simulink model "ctrl_studentmclab"  (R2015a)
settings: Solver=ode4  StartTime=0.0  StopTime=inf  FixedStep=0.01  RelTol=1e-3
(part 3 of 3)

== system ctrl_studentmclab/Observer/eta_hat_ut ==
  In1 : Inport
  Demux1 : Demux  Outputs=3
  psi_hat : S-Function  Priority=1  FunctionName=NIVeriStandIO  Parameters=width dtype portnum stime stype btype  mask(NI VeriStand Outport){portnum=1, width=-1, stime=-1, dtype=auto, stype=auto, btype=0}
      mask prompts: portnum "Port number:"; width "Port dimensions (-1 for dynamically sized):"; stime "Sample time (-1 for inherited):"; dtype "Data type:"; stype "Signal type:"; btype "Block type:"
      mask help: Use this outport on any level of nested subsystems to allow NI VeriStand software to map signals to it.
      mask init:
      | NIVeriStandIO_init;
      settings: CopyFcn=NIVeriStand_MDL_functions('', 'IO_copy');  DeleteFcn=NIVeriStand_MDL_functions('', 'IO_delete');  MoveFcn=set_param(gcb, 'Mask', 'on');
      mask Callback portnum: NIVeriStand_MDL_functions('', 'IO_setportnum');
      mask TypeOptions dtype: auto | double | single | int8 | uint8 | int16 | uint16 | int32 | uint32 | boolean
      mask Callback dtype: NIVeriStand_MDL_functions('', 'IO_booleansignal');
      mask TypeOptions stype: auto | real | complex
      mask Display:
      | patch([-x x], [-y y], [.90980 .81960 .32156]);
      | plot([xrad -x x xrad], [yrad -y y yrad]);
      | fprintf('NI Out%d', portnum);
  x_hat : S-Function  Priority=2  FunctionName=NIVeriStandIO  Parameters=width dtype portnum stime stype btype  mask(NI VeriStand Outport){portnum=2, width=-1, stime=-1, dtype=auto, stype=auto, btype=0}
      mask prompts: portnum "Port number:"; width "Port dimensions (-1 for dynamically sized):"; stime "Sample time (-1 for inherited):"; dtype "Data type:"; stype "Signal type:"; btype "Block type:"
      mask help: Use this outport on any level of nested subsystems to allow NI VeriStand software to map signals to it.
      mask init:
      | NIVeriStandIO_init;
      settings: CopyFcn=NIVeriStand_MDL_functions('', 'IO_copy');  DeleteFcn=NIVeriStand_MDL_functions('', 'IO_delete');  MoveFcn=set_param(gcb, 'Mask', 'on');
      mask Callback portnum: NIVeriStand_MDL_functions('', 'IO_setportnum');
      mask TypeOptions dtype: auto | double | single | int8 | uint8 | int16 | uint16 | int32 | uint32 | boolean
      mask Callback dtype: NIVeriStand_MDL_functions('', 'IO_booleansignal');
      mask TypeOptions stype: auto | real | complex
      mask Display:
      | patch([-x x], [-y y], [.90980 .81960 .32156]);
      | plot([xrad -x x xrad], [yrad -y y yrad]);
      | fprintf('NI Out%d', portnum);
  y_hat : S-Function  Priority=3  FunctionName=NIVeriStandIO  Parameters=width dtype portnum stime stype btype  mask(NI VeriStand Outport){portnum=3, width=-1, stime=-1, dtype=auto, stype=auto, btype=0}
      mask prompts: portnum "Port number:"; width "Port dimensions (-1 for dynamically sized):"; stime "Sample time (-1 for inherited):"; dtype "Data type:"; stype "Signal type:"; btype "Block type:"
      mask help: Use this outport on any level of nested subsystems to allow NI VeriStand software to map signals to it.
      mask init:
      | NIVeriStandIO_init;
      settings: CopyFcn=NIVeriStand_MDL_functions('', 'IO_copy');  DeleteFcn=NIVeriStand_MDL_functions('', 'IO_delete');  MoveFcn=set_param(gcb, 'Mask', 'on');
      mask Callback portnum: NIVeriStand_MDL_functions('', 'IO_setportnum');
      mask TypeOptions dtype: auto | double | single | int8 | uint8 | int16 | uint16 | int32 | uint32 | boolean
      mask Callback dtype: NIVeriStand_MDL_functions('', 'IO_booleansignal');
      mask TypeOptions stype: auto | real | complex
      mask Display:
      | patch([-x x], [-y y], [.90980 .81960 .32156]);
      | plot([xrad -x x xrad], [yrad -y y yrad]);
      | fprintf('NI Out%d', portnum);
  wires:
  Demux1/3 -> psi_hat/1
  Demux1/1 -> x_hat/1
  Demux1/2 -> y_hat/1
  In1/1 -> Demux1/1

== system ctrl_studentmclab/Observer/nu_hat_ut ==
  In1 : Inport
  Demux1 : Demux  Outputs=3
  r_hat : S-Function  Priority=1  FunctionName=NIVeriStandIO  Parameters=width dtype portnum stime stype btype  mask(NI VeriStand Outport){portnum=1, width=-1, stime=-1, dtype=auto, stype=auto, btype=0}
      mask prompts: portnum "Port number:"; width "Port dimensions (-1 for dynamically sized):"; stime "Sample time (-1 for inherited):"; dtype "Data type:"; stype "Signal type:"; btype "Block type:"
      mask help: Use this outport on any level of nested subsystems to allow NI VeriStand software to map signals to it.
      mask init:
      | NIVeriStandIO_init;
      settings: CopyFcn=NIVeriStand_MDL_functions('', 'IO_copy');  DeleteFcn=NIVeriStand_MDL_functions('', 'IO_delete');  MoveFcn=set_param(gcb, 'Mask', 'on');
      mask Callback portnum: NIVeriStand_MDL_functions('', 'IO_setportnum');
      mask TypeOptions dtype: auto | double | single | int8 | uint8 | int16 | uint16 | int32 | uint32 | boolean
      mask Callback dtype: NIVeriStand_MDL_functions('', 'IO_booleansignal');
      mask TypeOptions stype: auto | real | complex
      mask Display:
      | patch([-x x], [-y y], [.90980 .81960 .32156]);
      | plot([xrad -x x xrad], [yrad -y y yrad]);
      | fprintf('NI Out%d', portnum);
  u_hat : S-Function  Priority=2  FunctionName=NIVeriStandIO  Parameters=width dtype portnum stime stype btype  mask(NI VeriStand Outport){portnum=2, width=-1, stime=-1, dtype=auto, stype=auto, btype=0}
      mask prompts: portnum "Port number:"; width "Port dimensions (-1 for dynamically sized):"; stime "Sample time (-1 for inherited):"; dtype "Data type:"; stype "Signal type:"; btype "Block type:"
      mask help: Use this outport on any level of nested subsystems to allow NI VeriStand software to map signals to it.
      mask init:
      | NIVeriStandIO_init;
      settings: CopyFcn=NIVeriStand_MDL_functions('', 'IO_copy');  DeleteFcn=NIVeriStand_MDL_functions('', 'IO_delete');  MoveFcn=set_param(gcb, 'Mask', 'on');
      mask Callback portnum: NIVeriStand_MDL_functions('', 'IO_setportnum');
      mask TypeOptions dtype: auto | double | single | int8 | uint8 | int16 | uint16 | int32 | uint32 | boolean
      mask Callback dtype: NIVeriStand_MDL_functions('', 'IO_booleansignal');
      mask TypeOptions stype: auto | real | complex
      mask Display:
      | patch([-x x], [-y y], [.90980 .81960 .32156]);
      | plot([xrad -x x xrad], [yrad -y y yrad]);
      | fprintf('NI Out%d', portnum);
  v_hat : S-Function  Priority=3  FunctionName=NIVeriStandIO  Parameters=width dtype portnum stime stype btype  mask(NI VeriStand Outport){portnum=3, width=-1, stime=-1, dtype=auto, stype=auto, btype=0}
      mask prompts: portnum "Port number:"; width "Port dimensions (-1 for dynamically sized):"; stime "Sample time (-1 for inherited):"; dtype "Data type:"; stype "Signal type:"; btype "Block type:"
      mask help: Use this outport on any level of nested subsystems to allow NI VeriStand software to map signals to it.
      mask init:
      | NIVeriStandIO_init;
      settings: CopyFcn=NIVeriStand_MDL_functions('', 'IO_copy');  DeleteFcn=NIVeriStand_MDL_functions('', 'IO_delete');  MoveFcn=set_param(gcb, 'Mask', 'on');
      mask Callback portnum: NIVeriStand_MDL_functions('', 'IO_setportnum');
      mask TypeOptions dtype: auto | double | single | int8 | uint8 | int16 | uint16 | int32 | uint32 | boolean
      mask Callback dtype: NIVeriStand_MDL_functions('', 'IO_booleansignal');
      mask TypeOptions stype: auto | real | complex
      mask Display:
      | patch([-x x], [-y y], [.90980 .81960 .32156]);
      | plot([xrad -x x xrad], [yrad -y y yrad]);
      | fprintf('NI Out%d', portnum);
  wires:
  Demux1/3 -> r_hat/1
  Demux1/1 -> u_hat/1
  Demux1/2 -> v_hat/1
  In1/1 -> Demux1/1

== system ctrl_studentmclab/tau to real ship (only use in MCLab)/To thruster of real ship ==
  u to thrusters : Inport
  control input u exceeds bounds : S-Function  Priority=8  FunctionName=NIVeriStandIO  Parameters=width dtype portnum stime stype btype  mask(NI VeriStand Outport){portnum=8, width=-1, stime=-1, dtype=auto, stype=auto, btype=0}
      mask prompts: portnum "Port number:"; width "Port dimensions (-1 for dynamically sized):"; stime "Sample time (-1 for inherited):"; dtype "Data type:"; stype "Signal type:"; btype "Block type:"
      mask help: Use this outport on any level of nested subsystems to allow NI VeriStand software to map signals to it.
      mask init:
      | NIVeriStandIO_init;
      settings: CopyFcn=NIVeriStand_MDL_functions('', 'IO_copy');  DeleteFcn=NIVeriStand_MDL_functions('', 'IO_delete');  MoveFcn=set_param(gcb, 'Mask', 'on');
      mask Callback portnum: NIVeriStand_MDL_functions('', 'IO_setportnum');
      mask TypeOptions dtype: auto | double | single | int8 | uint8 | int16 | uint16 | int32 | uint32 | boolean
      mask Callback dtype: NIVeriStand_MDL_functions('', 'IO_booleansignal');
      mask TypeOptions stype: auto | real | complex
      mask Display:
      | patch([-x x], [-y y], [.90980 .81960 .32156]);
      | plot([xrad -x x xrad], [yrad -y y yrad]);
      | fprintf('NI Out%d', portnum);
  control limit checking : MATLAB Function  TreatAsAtomicUnit=on
  u : Subsystem
  wires:
  control limit checking/1(fault) -> control input u exceeds bounds/1
  u to thrusters/1 -> control limit checking/1(u), u/1(u)

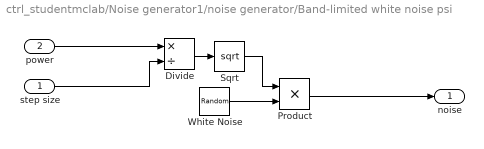
== system ctrl_studentmclab/Noise generator1/noise generator/Band-limited white noise psi ==
  step size : Inport
  power : Inport  Port=2
  Divide : Product  Inputs=*/
  Product : Product
  Sqrt : Sqrt  SaturateOnIntegerOverflow=on
  White Noise : RandomNumber  DisableCoverage=on  Seed=9025
  noise : Outport
  wires:
  White Noise/1 -> Product/2
  Product/1 -> noise/1
  step size/1 -> Divide/2
  Divide/1 -> Sqrt/1
  Sqrt/1 -> Product/1
  power/1 -> Divide/1

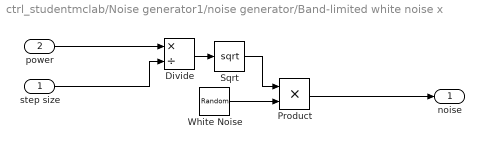
== system ctrl_studentmclab/Noise generator1/noise generator/Band-limited white noise x ==
  step size : Inport
  power : Inport  Port=2
  Divide : Product  Inputs=*/
  Product : Product
  Sqrt : Sqrt  SaturateOnIntegerOverflow=on
  White Noise : RandomNumber  DisableCoverage=on  Seed=9024
  noise : Outport
  wires:
  White Noise/1 -> Product/2
  Product/1 -> noise/1
  step size/1 -> Divide/2
  Divide/1 -> Sqrt/1
  Sqrt/1 -> Product/1
  power/1 -> Divide/1

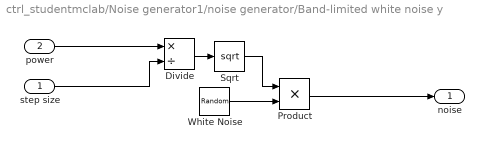
== system ctrl_studentmclab/Noise generator1/noise generator/Band-limited white noise y ==
  step size : Inport
  power : Inport  Port=2
  Divide : Product  Inputs=*/
  Product : Product
  Sqrt : Sqrt  SaturateOnIntegerOverflow=on
  White Noise : RandomNumber  DisableCoverage=on  Seed=123
  noise : Outport
  wires:
  White Noise/1 -> Product/2
  Product/1 -> noise/1
  step size/1 -> Divide/2
  Divide/1 -> Sqrt/1
  Sqrt/1 -> Product/1
  power/1 -> Divide/1

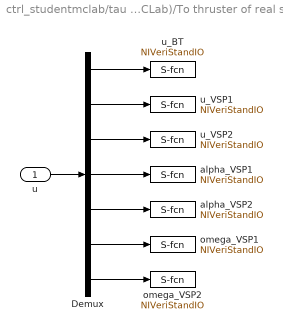
== system ctrl_studentmclab/tau to real ship (only use in MCLab)/To thruster of real ship/u ==
  u : Inport
  Demux : Demux  Outputs=7
  alpha_VSP1 : S-Function  Priority=4  FunctionName=NIVeriStandIO  Parameters=width dtype portnum stime stype btype  mask(NI VeriStand Outport){portnum=4, width=-1, stime=-1, dtype=auto, stype=auto, btype=0}
      mask prompts: portnum "Port number:"; width "Port dimensions (-1 for dynamically sized):"; stime "Sample time (-1 for inherited):"; dtype "Data type:"; stype "Signal type:"; btype "Block type:"
      mask help: Use this outport on any level of nested subsystems to allow NI VeriStand software to map signals to it.
      mask init:
      | NIVeriStandIO_init;
      settings: CopyFcn=NIVeriStand_MDL_functions('', 'IO_copy');  DeleteFcn=NIVeriStand_MDL_functions('', 'IO_delete');  MoveFcn=set_param(gcb, 'Mask', 'on');
      mask Callback portnum: NIVeriStand_MDL_functions('', 'IO_setportnum');
      mask TypeOptions dtype: auto | double | single | int8 | uint8 | int16 | uint16 | int32 | uint32 | boolean
      mask Callback dtype: NIVeriStand_MDL_functions('', 'IO_booleansignal');
      mask TypeOptions stype: auto | real | complex
      mask Display:
      | patch([-x x], [-y y], [.90980 .81960 .32156]);
      | plot([xrad -x x xrad], [yrad -y y yrad]);
      | fprintf('NI Out%d', portnum);
  alpha_VSP2 : S-Function  Priority=1  FunctionName=NIVeriStandIO  Parameters=width dtype portnum stime stype btype  mask(NI VeriStand Outport){portnum=1, width=-1, stime=-1, dtype=auto, stype=auto, btype=0}
      mask prompts: portnum "Port number:"; width "Port dimensions (-1 for dynamically sized):"; stime "Sample time (-1 for inherited):"; dtype "Data type:"; stype "Signal type:"; btype "Block type:"
      mask help: Use this outport on any level of nested subsystems to allow NI VeriStand software to map signals to it.
      mask init:
      | NIVeriStandIO_init;
      settings: CopyFcn=NIVeriStand_MDL_functions('', 'IO_copy');  DeleteFcn=NIVeriStand_MDL_functions('', 'IO_delete');  MoveFcn=set_param(gcb, 'Mask', 'on');
      mask Callback portnum: NIVeriStand_MDL_functions('', 'IO_setportnum');
      mask TypeOptions dtype: auto | double | single | int8 | uint8 | int16 | uint16 | int32 | uint32 | boolean
      mask Callback dtype: NIVeriStand_MDL_functions('', 'IO_booleansignal');
      mask TypeOptions stype: auto | real | complex
      mask Display:
      | patch([-x x], [-y y], [.90980 .81960 .32156]);
      | plot([xrad -x x xrad], [yrad -y y yrad]);
      | fprintf('NI Out%d', portnum);
  omega_VSP1 : S-Function  Priority=2  FunctionName=NIVeriStandIO  Parameters=width dtype portnum stime stype btype  mask(NI VeriStand Outport){portnum=2, width=-1, stime=-1, dtype=auto, stype=auto, btype=0}
      mask prompts: portnum "Port number:"; width "Port dimensions (-1 for dynamically sized):"; stime "Sample time (-1 for inherited):"; dtype "Data type:"; stype "Signal type:"; btype "Block type:"
      mask help: Use this outport on any level of nested subsystems to allow NI VeriStand software to map signals to it.
      mask init:
      | NIVeriStandIO_init;
      settings: CopyFcn=NIVeriStand_MDL_functions('', 'IO_copy');  DeleteFcn=NIVeriStand_MDL_functions('', 'IO_delete');  MoveFcn=set_param(gcb, 'Mask', 'on');
      mask Callback portnum: NIVeriStand_MDL_functions('', 'IO_setportnum');
      mask TypeOptions dtype: auto | double | single | int8 | uint8 | int16 | uint16 | int32 | uint32 | boolean
      mask Callback dtype: NIVeriStand_MDL_functions('', 'IO_booleansignal');
      mask TypeOptions stype: auto | real | complex
      mask Display:
      | patch([-x x], [-y y], [.90980 .81960 .32156]);
      | plot([xrad -x x xrad], [yrad -y y yrad]);
      | fprintf('NI Out%d', portnum);
  omega_VSP2 : S-Function  Priority=3  FunctionName=NIVeriStandIO  Parameters=width dtype portnum stime stype btype  mask(NI VeriStand Outport){portnum=3, width=-1, stime=-1, dtype=auto, stype=auto, btype=0}
      mask prompts: portnum "Port number:"; width "Port dimensions (-1 for dynamically sized):"; stime "Sample time (-1 for inherited):"; dtype "Data type:"; stype "Signal type:"; btype "Block type:"
      mask help: Use this outport on any level of nested subsystems to allow NI VeriStand software to map signals to it.
      mask init:
      | NIVeriStandIO_init;
      settings: CopyFcn=NIVeriStand_MDL_functions('', 'IO_copy');  DeleteFcn=NIVeriStand_MDL_functions('', 'IO_delete');  MoveFcn=set_param(gcb, 'Mask', 'on');
      mask Callback portnum: NIVeriStand_MDL_functions('', 'IO_setportnum');
      mask TypeOptions dtype: auto | double | single | int8 | uint8 | int16 | uint16 | int32 | uint32 | boolean
      mask Callback dtype: NIVeriStand_MDL_functions('', 'IO_booleansignal');
      mask TypeOptions stype: auto | real | complex
      mask Display:
      | patch([-x x], [-y y], [.90980 .81960 .32156]);
      | plot([xrad -x x xrad], [yrad -y y yrad]);
      | fprintf('NI Out%d', portnum);
  u_BT : S-Function  Priority=5  FunctionName=NIVeriStandIO  Parameters=width dtype portnum stime stype btype  mask(NI VeriStand Outport){portnum=5, width=-1, stime=-1, dtype=auto, stype=auto, btype=0}
      mask prompts: portnum "Port number:"; width "Port dimensions (-1 for dynamically sized):"; stime "Sample time (-1 for inherited):"; dtype "Data type:"; stype "Signal type:"; btype "Block type:"
      mask help: Use this outport on any level of nested subsystems to allow NI VeriStand software to map signals to it.
      mask init:
      | NIVeriStandIO_init;
      settings: CopyFcn=NIVeriStand_MDL_functions('', 'IO_copy');  DeleteFcn=NIVeriStand_MDL_functions('', 'IO_delete');  MoveFcn=set_param(gcb, 'Mask', 'on');
      mask Callback portnum: NIVeriStand_MDL_functions('', 'IO_setportnum');
      mask TypeOptions dtype: auto | double | single | int8 | uint8 | int16 | uint16 | int32 | uint32 | boolean
      mask Callback dtype: NIVeriStand_MDL_functions('', 'IO_booleansignal');
      mask TypeOptions stype: auto | real | complex
      mask Display:
      | patch([-x x], [-y y], [.90980 .81960 .32156]);
      | plot([xrad -x x xrad], [yrad -y y yrad]);
      | fprintf('NI Out%d', portnum);
  u_VSP1 : S-Function  Priority=6  FunctionName=NIVeriStandIO  Parameters=width dtype portnum stime stype btype  mask(NI VeriStand Outport){portnum=6, width=-1, stime=-1, dtype=auto, stype=auto, btype=0}
      mask prompts: portnum "Port number:"; width "Port dimensions (-1 for dynamically sized):"; stime "Sample time (-1 for inherited):"; dtype "Data type:"; stype "Signal type:"; btype "Block type:"
      mask help: Use this outport on any level of nested subsystems to allow NI VeriStand software to map signals to it.
      mask init:
      | NIVeriStandIO_init;
      settings: CopyFcn=NIVeriStand_MDL_functions('', 'IO_copy');  DeleteFcn=NIVeriStand_MDL_functions('', 'IO_delete');  MoveFcn=set_param(gcb, 'Mask', 'on');
      mask Callback portnum: NIVeriStand_MDL_functions('', 'IO_setportnum');
      mask TypeOptions dtype: auto | double | single | int8 | uint8 | int16 | uint16 | int32 | uint32 | boolean
      mask Callback dtype: NIVeriStand_MDL_functions('', 'IO_booleansignal');
      mask TypeOptions stype: auto | real | complex
      mask Display:
      | patch([-x x], [-y y], [.90980 .81960 .32156]);
      | plot([xrad -x x xrad], [yrad -y y yrad]);
      | fprintf('NI Out%d', portnum);
  u_VSP2 : S-Function  Priority=7  FunctionName=NIVeriStandIO  Parameters=width dtype portnum stime stype btype  mask(NI VeriStand Outport){portnum=7, width=-1, stime=-1, dtype=auto, stype=auto, btype=0}
      mask prompts: portnum "Port number:"; width "Port dimensions (-1 for dynamically sized):"; stime "Sample time (-1 for inherited):"; dtype "Data type:"; stype "Signal type:"; btype "Block type:"
      mask help: Use this outport on any level of nested subsystems to allow NI VeriStand software to map signals to it.
      mask init:
      | NIVeriStandIO_init;
      settings: CopyFcn=NIVeriStand_MDL_functions('', 'IO_copy');  DeleteFcn=NIVeriStand_MDL_functions('', 'IO_delete');  MoveFcn=set_param(gcb, 'Mask', 'on');
      mask Callback portnum: NIVeriStand_MDL_functions('', 'IO_setportnum');
      mask TypeOptions dtype: auto | double | single | int8 | uint8 | int16 | uint16 | int32 | uint32 | boolean
      mask Callback dtype: NIVeriStand_MDL_functions('', 'IO_booleansignal');
      mask TypeOptions stype: auto | real | complex
      mask Display:
      | patch([-x x], [-y y], [.90980 .81960 .32156]);
      | plot([xrad -x x xrad], [yrad -y y yrad]);
      | fprintf('NI Out%d', portnum);
  wires:
  u/1 -> Demux/1
  Demux/1 -> u_BT/1
  Demux/2 -> u_VSP1/1
  Demux/3 -> u_VSP2/1
  Demux/4 -> alpha_VSP1/1
  Demux/5 -> alpha_VSP2/1
  Demux/6 -> omega_VSP1/1
  Demux/7 -> omega_VSP2/1

== matlab function ctrl_studentmclab/tau to real ship (only use in MCLab)/Full thrust allocation ==
  data: X_d input; Y_d input; u_BT output; N_d input; u_VSP output; alpha_VSP output; VSP_on input; omega_VSP output
function [u_BT,u_VSP,alpha_VSP,omega_VSP]= fcn(X_d,Y_d,N_d, VSP_on)

% Forces and moments vector
tau = [X_d
       Y_d
       N_d];

% Extended thrust configuration matrix
l_VSP = -0.4575;
l_BT  = 0.3875;
T = [1 0     0
     0 1     1
     0 l_VSP l_BT];

% Extended thrust coefficient matrix
F_max_VSP = 1.165;
F_max_BT  = 2.629;
K = [F_max_VSP 0         0
     0         F_max_VSP 0
     0         0         F_max_BT];

% tau = T*K*u inverse
u = K\(T\tau);

u_BT      = u(3);

u_VSP_x   = u(1);
u_VSP_y   = u(2);
u_VSP     = sqrt(u_VSP_x^2 + u_VSP_y^2);
alpha_VSP = atan2(u_VSP_y,u_VSP_x);

if VSP_on
    omega_VSP = 0.3;
else
    omega_VSP = 0;
end

== matlab function ctrl_studentmclab/tau to real ship (only use in MCLab)/To thruster of real ship/control limit checking ==
  data: u input; fault output
function fault= fcn(u)
u_BT       = u(1);
u_VSP1     = u(2);
u_VSP2     = u(3);
alpha_VSP1 = u(4);
alpha_VSP2 = u(5);
omega_VSP1 = u(6);
omega_VSP2 = u(7);

OK = -1  <= u_BT       & u_BT       <= 1  & ...
     0   <= u_VSP1     & u_VSP1     <= 1  & ...
     0   <= u_VSP2     & u_VSP2     <= 1  & ...
     -pi <= alpha_VSP1 & alpha_VSP1 <= pi & ...
     -pi <= alpha_VSP2 & alpha_VSP2 <= pi & ...
     -1  <= omega_VSP1 & omega_VSP1 <= 1  & ...
     -1  <= omega_VSP2 & omega_VSP2 <= 1  ;
 
fault = ~OK;

== matlab function ctrl_studentmclab/tau to real ship (only use in MCLab)/Limited allocation: VSP only  in surge and BT only in yaw ==
  data: X_VSP input; u_BT output; N_BT input; u_VSP output; alpha_VSP output; omega_VSP output
function [u_BT,u_VSP,alpha_VSP,omega_VSP]= fcn(X_VSP,N_BT)

l_BT     = 0.3875;
F_max_BT = 2.629;
u_BT     = N_BT/(l_BT*F_max_BT);

omega_VSP = 0.3;
F_max_VSP = 1.165;
u_VSP     = abs(X_VSP)/(2*F_max_VSP);
alpha_VSP = pi*(X_VSP<=0); % 0 if positive X_VSP, pi if negative

== matlab function ctrl_studentmclab/Noise generator1/Downsample	signal/MATLAB Function ==
  data: f input; h input; i input; count output
function count = fcn(f,h,i)
%#codegen
sampling_time = 1/f;
if (i+1)*h >= sampling_time
    count = 0;
else
    count = i+1;
end

== matlab function ctrl_studentmclab/Noise generator1/Sample & hold/MATLAB Function1 ==
  data: counter input; input input; hold input; output output
function output = fcn(counter,input,hold)
%#codegen

if counter == 0
    output = input;
else
    output = hold;
end

== matlab function ctrl_studentmclab/Observer/D ==
  data: nu input; D output
function D = fcn(nu)

d11 = 0.6555-0.354*abs(nu(1))+3.787*(nu(1))^2; 
d22 = 1.33+2.776*abs(nu(2))+64.91*(nu(2))^2+0.805*abs(nu(3)) ; 
d23 = 7.25+0.845*abs(nu(2))+3.45*abs(nu(3));
d32 = 0.2088*abs(nu(2))-0.130*abs(nu(3));
d33 = 1.9-0.08*abs(nu(2))+0.75*abs(nu(3));

D=[d11 0    0
   0   d22  d23
   0   d32  d33];

== matlab function ctrl_studentmclab/Observer/L1/MATLAB Function ==
  data: u input; y output
function y = fcn(u)
y = diag([u(1),u(2),u(3)]);

== matlab function ctrl_studentmclab/DP-system/Ellipsoidal path ==
  data: s input; c input; eta_v output size=11; r input; U_ref input; psi input
function eta_v = fcn(s,c,r,U_ref,psi)

eta_d = [c(1) + r(1)*cos(2*pi*s)
         c(2) + r(2)*sin(2*pi*s)
         atan2(-r(2)*cos(2*pi*s),r(1)*sin(2*pi*s))];

%wrapping psi_d     
persistent k;
k=0;				

if abs((eta_d(3)+(2*pi*k))-(psi)) > pi
   if (psi) < eta_d(3)+(2*pi*k)
       k = k-1;
   elseif (psi) > eta_d(3)+(2*pi*k)
       k = k+1;
   end
end 
eta_d(3)=eta_d(3)+(2*pi*k);
     
     
eta_ds = 2*pi*[-r(1)*sin(2*pi*s)
                r(2)*cos(2*pi*s)
               (-r(1)*r(2))/(r(2)^2*cos(2*pi*s)^2 + r(1)^2*sin(2*pi*s)^2)];

eta_dss = (2*pi)^2*[-r(1)*cos(2*pi*s)
                     -r(2)*sin(2*pi*s)
                     (4*r(2)*r(1)*(r(2)^2 - r(1)^2)*sin(2*2*pi*s))/(r(2)^2 + r(1)^2 + r(2)^2*cos(2*2*pi*s) - r(1)^2*cos(2*2*pi*s))^2];
     
     
U_s = U_ref/(sqrt(r(1)^2 * sin(2*pi*s)^2 + r(2)^2 * cos(2*pi*s)^2));

U_ss = -U_ref*(r(1)^2*sin(2*pi*s)*(2*pi)^3*cos(2*pi*s)-r(2)^2*cos(2*pi*s)*(2*pi)^3*sin(2*pi*s))/...
    ((2*pi*-r(1)*sin(2*pi*s))^2 + (r(2)*cos(2*pi*s)*2*pi)^2)^1.5;

eta_v = [eta_d; eta_ds; eta_dss ; U_s; U_ss];

== matlab function ctrl_studentmclab/Observer/L2/MATLAB Function ==
  data: u input; y output
function y = fcn(u)
y = diag([u(1),u(2),u(3)]);

== matlab function ctrl_studentmclab/DP-system/controller ==
  data: z1 input; z2 input; s_dot input; a_1 output; eta_v input; nu input; tau output; Kd input; D1 output; z11 output; ma output; Kdz output
function [a_1, tau,D1,z11,ma,Kdz] = fcn(z1,z2,s_dot,eta_v,nu,Kd)
%Kinetics
u   = nu(1);
v   = nu(2);
r   = nu(3);
% MATRICES
m    = 14.79;   
I_z  =  1.76;  
x_g = 0.0375;       
% Added mass
X_ud  =     -2.0;						% Table B.1
Y_vd =     -1.0;	N_vd =    -0.0;		% Table B.1 guestimate
Y_rd =      -0.0;	N_rd =    -1.0;		% Table B.1

% Total mass matrix
m_11 = m-X_ud;
m_22 = m-Y_vd;
m_23 = m*x_g-Y_rd;
m_32 = m*x_g-N_vd;
m_33 = I_z-N_rd;

M    = [m_11 0    0
        0    m_22 m_23
        0    m_32 m_33];
	
% Damping coefficients
% Comments at the end of the lines indicate the old values used.
X_u		= -0.6555;		X_v		= 0;
X_uu 	= 0.3545;		X_vv	= -2.443;
X_uuu 	= -3.787;		X_vvv	= 0;
Y_v		= -1.33;    	Y_r		= -7.250; % Y_r
Y_vv	= -2.776;		Y_rr	= -3.450; % Y_rr
Y_vvv	= -64.91;		Y_rrr	= 0;
Y_rv	= -0.805;		Y_vr	= -0.845; % Y_rv, Y_vr
N_v		= 0;			N_r		= -1.900; % N_r
N_vv	= -0.2088;		N_rr	= -0.750; % N_rr
N_vvv	= 0;			N_rrr	= 0;
N_rv	= 0.130;		N_vr	= 0.080; % N_rv, N_vr

% Correolis matrix
c_13 = -(m-Y_vd)*v-(m*x_g-Y_rd)*r;
c_23 = (m-X_ud)*u;
C    = [0     0     c_13
        0     0     c_23
        -c_13 -c_23 0   ];

% Assembly of the damping matrix
d_11 = -X_u - X_uu*u - X_uuu*u^2;
d_22 = -Y_v - Y_vv*v - Y_vvv*v^2 - Y_rv*abs(r);
d_33 = -N_r - N_rr*abs(r) - N_rrr*r^2 - N_vr*abs(v); % using abs(r)

d_12 = -X_v - X_vv*v - X_vvv*v^2;
d_23 = -Y_r - Y_rr*abs(r) - Y_rrr*r^2 - Y_vr*abs(v);
d_32 = -N_v - N_vv*v - N_vvv*v^2 - N_rv*abs(r);

D    = [d_11 d_12 0
        0    d_22 d_23
        0    d_32 d_33];

    

%Eta_d derivatives and U_s
eta     = eta_v(1:3);
eta_ds  = eta_v(4:6);
eta_dss = eta_v(7:9);
U_s     = eta_v(10);
U_ss    = eta_v(11);
%Rotation matrix and derivative
R = [cos(eta(3)) -sin(eta(3)) 0
     sin(eta(3))  cos(eta(3)) 0
     0            0           1];
 
S = [0     -eta(3) 0
     eta(3)   0    0
     0        0    0]; 
 
%Gain matrices 
Kp = diag([0.2,0.2,0.1]);
%Kd = diag([25 15 30]);

%Controller alpha 1
a_1 = -Kp*z1 +R'*eta_ds*U_s;


%Alpha derivative
a_t = -Kp*(-S*z1+nu)-S*R'*eta_ds*U_s;
a_s = -Kp*R'*eta_ds+R'*eta_dss*U_s+R'*eta_ds*U_ss;
a_dot = a_t + a_s.*s_dot;

%Controller tau - C removed
tau = D*nu- z1 + M*a_dot - Kd*z2;
D1 = D*nu;
z11 = z1;
ma = M*a_dot;
Kdz = Kd*z2;
%tau = a_1;
%tau = [tau(1);tau(2);tau(3)];

== matlab function ctrl_studentmclab/DP-system/Straight -line  ==
  data: eta_0 input; eta_1 input; U_ref input; eta_v output size=11; s input
function eta_v = fcn(eta_0,eta_1,U_ref,s)

eta_d = [(eta_1(1)-eta_0(1))*s + eta_0(1)
         (eta_1(2)-eta_0(2))*s + eta_0(2) 
         atan((eta_1(2)-eta_0(2))/(eta_1(1)-eta_0(1)))];
     
eta_ds = [(eta_1(1)-eta_0(1))
          (eta_1(2)-eta_0(2))
          0];
eta_dss = [0; 0; 0];



     
U_s = U_ref / sqrt((eta_1(1)-eta_0(1))^2 + (eta_1(2)-eta_0(2))^2);

U_ss = 0;

 
eta_v = [eta_d; eta_ds; eta_dss ; U_s; U_ss];

== matlab function ctrl_studentmclab/DP-system/update law ==
  data: eta input; eta_v input; z1 input; my input; s_dot1 output size=1; temp input; i output
function [s_dot1,i] = fcn(eta,eta_v,z1,my,temp)

i = temp(1); 
s = temp(3); 
s_dot1 = temp(2);
%Getting vectors
eta_d   = eta_v(1:3);
eta_ds  = eta_v(4:6);
eta_dss = eta_v(7:9);
U_s     = eta_v(10);


R = [cos(eta(3)) -sin(eta(3)) 0
     sin(eta(3))  cos(eta(3)) 0
     0            0           1];

V1_s = -z1'*R'*eta_ds;



    s_dot1 = U_s - (my/norm(eta_ds))*V1_s;

if i == 0 
    
    if s > 1;
        i = 1; 
    end 
end 

if i == 1
    s_dot1 = -(U_s - (my/norm(eta_ds))*V1_s); 
    if s < 0;
        i = 0; 
    end 
end

== matlab function ctrl_studentmclab/DP-system/z1//z2 ==
  data: eta_v input; z1 output; eta input; nu input; alpha input; z2 output
function [z1,z2]  = fcn(eta_v,eta,nu,alpha)


eta_d1 = [eta_v(1);eta_v(2);eta_v(3)];
eta1 = [eta(1);eta(2);eta(3)];

R = [cos(eta(3)) -sin(eta(3)) 0
     sin(eta(3))  cos(eta(3)) 0
     0            0           1];
 
 z1 = R'*(eta1-eta_d1);
 
 z2 = nu - alpha;

== matlab function ctrl_studentmclab/Observer/L3/MATLAB Function ==
  data: u input; y output
function y = fcn(u)
y = diag([u(1),u(2),u(3)]);

== matlab function ctrl_studentmclab/Observer/Rotation matrix ==
  data: psi input; R output; RT output
function [R,RT] = fcn(psi)
R=[ cos(psi) -sin(psi) 0
    sin(psi) cos(psi)  0
    0        0         1];

RT=R';

== matlab function ctrl_studentmclab/DP-system/signal switch  ==
  data: straight input; signal output; swich input; ellipse input
function signal = fcn(straight,swich,ellipse)

signal = straight; 
if swich == 1
    signal = straight;
end

if swich == 2
    signal = ellipse;
end

== matlab function ctrl_studentmclab/DP-system/Kd/MATLAB Function ==
  data: u input; y output
function y = fcn(u)
y = diag([u(1),u(2),u(3)]);

== matlab function ctrl_studentmclab/DP-system/inputs ==
  data: eta input; eta_0 output; eta_d output; U_ref_l output; r output; c output; U_ref_e output; my output; s input
function [eta_0,eta_d,U_ref_l,r,c,U_ref_e,my]  = fcn(eta,s)
% i = temp1(1);  
% U_ref_l = temp1(2); 
eta_0 = [2 0];
eta_d = [4 2]; 
r = [7 7]; 
c = [0 0];  
U_max = 0.5; 
my = 0; 
dp = 0; % my må være null hvis dp = 1
U_ref_l = U_max/5;
U_ref_e = 0.05;


% % ikke dp i starten
% 
%     if i == 0
%         U_ref_l = U_max/5; 
%         if s > 1;
%             i = 1; 
%         end 
%     end 
% 
%     if i == 1
%         U_ref_l = -U_max/5;
%         if s < 0
%             i = 0; 
%         end
%     end 
% U_ref = U_ref_l;
% 
% % error = [0 0];
% % error(1) = eta(1) - eta_0(1);
% % error(2) = eta(2) - eta_0(2); 
% % DP i starten
% % if dp == 1 
% % if i == 0 
% %     if (abs(error(1)) < 0.01 && abs(error(2)) < 0.01)
% %     U_ref_l = U_max/5;
% %     i = 1; 
% %     end
% % end 
% % 
% % if i == 1
% %     if s >= 1
% %         U_ref_l = -U_max/5;
% %         i = 2; 
% %     end     
% % end
% % 
% % if i == 2
% %     if s <= 0 
% %         U_ref_l = U_max/5; 
% %         i = 1; 
% %     end 
% % end 
% % end
% 
% temp = [0 0];
% temp(1) = i; 
% temp(2) = U_ref_l;

== matlab function ctrl_studentmclab/Switch joystick and DP-system ==
  data: guidance input; signal output; swich input; joystick input
%% Function that takes in impulse button sigals [0,1] and sends out a 
% different signal depentent pn which button has been pressed

function signal = fcn(guidance,swich,joystick)

signal = [0;0;0]; 
if swich == 1
    signal = guidance;
end

if swich == 2
    signal = guidance;
end

if swich == 3
    signal = joystick;
end

== matlab function ctrl_studentmclab/joystick1/MATLAB Function ==
  data: x input; u output; y input
function u = fcn(x,y)

if abs(x) > 5 || abs(y) > 5
    u = 1; %wtf fiks 
else 
    u = 1;
end

== matlab function ctrl_studentmclab/joystick1/Thrust allocation ==
  data: X input; Y input; u_BT output; N input; u_VSP output; alpha_VSP output; VSP_on input; omega_VSP output
function [u_BT,u_VSP,alpha_VSP,omega_VSP]= fcn(X,Y,N, VSP_on)

% Forces and moments vector
tau = [X
       Y
       N];

% Extended thrust configuration matrix
l_VSP = -0.4575;
l_BT  = 0.3875;
T = [1 0     0
     0 1     1
     0 l_VSP l_BT];

% Extended thrust coefficient matrix
F_max_VSP = 1.165;
F_max_BT  = 2.629;
K = [F_max_VSP 0         0
     0         F_max_VSP 0
     0         0         F_max_BT];

% tau = T*K*u inverse
u = (T*K)\tau;

u_BT      = u(3);

u_VSP_x   = u(1);
u_VSP_y   = u(2);
u_VSP     = sqrt(u_VSP_x^2 + u_VSP_y^2);
alpha_VSP = atan2(u_VSP_y,u_VSP_x);

if VSP_on
    omega_VSP = 0.3;
else
    omega_VSP = 0;
end

== matlab function ctrl_studentmclab/signal dropout check /MATLAB Function ==
  data: u input; y output; v input; vecx1 input; vecx output; vecy1 input; vecy output; d output
function [y,vecx,vecy,d] = fcn(u,v,vecx1,vecy1) 
vecx = vecx1;
vecy = vecy1;
for i = 2:10
vecx(i) = vecx(i-1);
vecy(i) = vecy(i-1);
end
vecx(1) = u(1);
vecy(1) = u(2); 

d = 1; 
if (numel(unique(vecx)) == 1 || numel(unique(vecy)) == 1)
    y = v; 
    d = 0;
else
    y = u;
end

== matlab function ctrl_studentmclab/switch/Switch_function ==
  data: arrows input; switch_signal output; temp input
%% Function that takes in impulse button sigals [0,1] and sends out a 
% different signal depentent pn which button has been pressed

function switch_signal = fcn(arrows,temp)
%#codegen
persistent signal;

signal = temp;

if arrows(1) ~= 0
    signal = 1;
end

if arrows(2) ~= 0
    signal = 2;
end

if arrows(3) ~= 0
    signal = 3;
end

switch_signal = signal;
